simulink model "servo_hub_task_sys"  (R2023a)
settings: Solver=FixedStepDiscrete  StartTime=0.0  StopTime=10.0  RelTol=1e-3
settings Model: Creator=Administrator  LastModifiedBy=Administrator

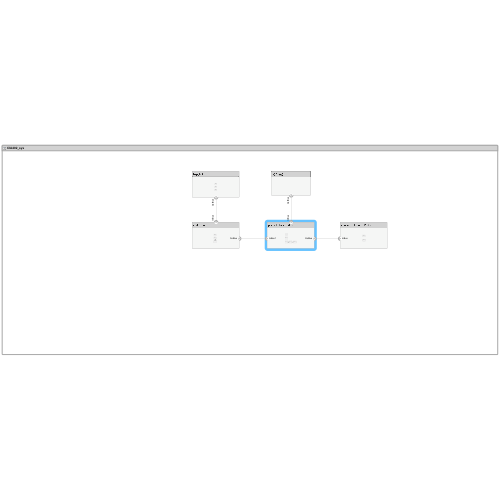
[thumbnail: Simulink's stored preview of the top-level diagram]
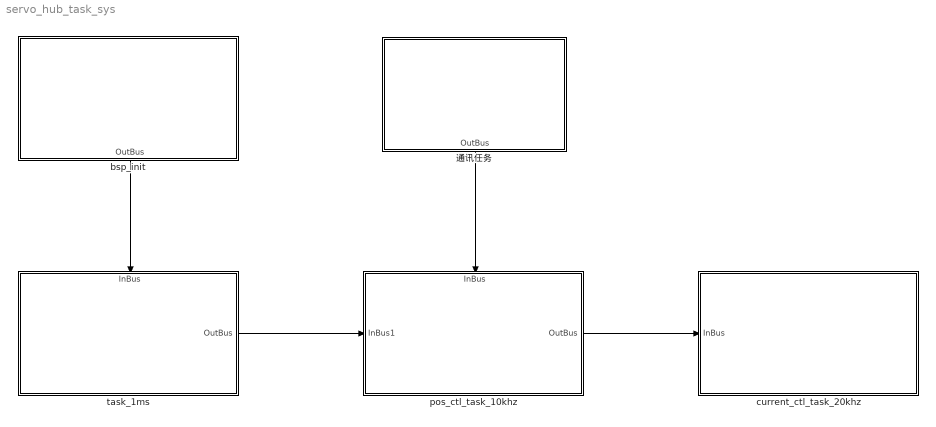
== system servo_hub_task_sys ==
  bsp_init : Subsystem
      settings: PortSchema="{\"entries\":[{\"content\":{\"headerSize\":26,\"margin\":15,\"minimumSpacing\":25,\"sides\":[{\"content\":{},\"type\":\"ConnectorPlacement.EquallySpacedRectSide\",\"uuid\":\"1beaa6a8-afd1-4db0-ba36-e52cb0b52ffd\"},{\"content\":{\"side\":\"RIGHT\"},\"type\":\"ConnectorPlacement.EquallySpacedRectSide\",\"uuid\":\"b483323e-58d5-432d-ab7d-aadce63dbe6f\"},{\"content\":{\"side\":\"TOP\"},\"type\":\"ConnectorPlacement.EquallySpacedRectSide\",\"uuid\":\"9aa6bb67-c79d-4421-a771-0f032b496522\"},{\"content\":{\"connectorIds\":[\"Out1\"],\"side\":\"BOTTOM\"},\"type\":\"ConnectorPlacement.EquallySpacedRectSide\",\"uuid\":\"df1d6553-7fe8-4c19-b309-8013b66b66f3\"}]},\"type\":\"ConnectorPlacement.EquallySpacedConnector\",\"uuid\":\"06545d34-e2f8-440d-8858-488d7d5d7ce4\"}],\"packageUris\":[\"http://schema.mathworks.com/mf0/Connector/R2020b\"],\"version\":\"1.0\"}"
  current_ctl_task_20khz : Subsystem
      settings: PortSchema="{\"entries\":[{\"content\":{\"headerSize\":26,\"margin\":15,\"minimumSpacing\":25,\"sides\":[{\"content\":{\"connectorIds\":[\"In1\"]},\"type\":\"ConnectorPlacement.EquallySpacedRectSide\",\"uuid\":\"1beaa6a8-afd1-4db0-ba36-e52cb0b52ffd\"},{\"content\":{\"side\":\"RIGHT\"},\"type\":\"ConnectorPlacement.EquallySpacedRectSide\",\"uuid\":\"b483323e-58d5-432d-ab7d-aadce63dbe6f\"},{\"content\":{\"side\":\"TOP\"},\"type\":\"ConnectorPlacement.EquallySpacedRectSide\",\"uuid\":\"9aa6bb67-c79d-4421-a771-0f032b496522\"}]},\"type\":\"ConnectorPlacement.EquallySpacedConnector\",\"uuid\":\"06545d34-e2f8-440d-8858-488d7d5d7ce4\"}],\"packageUris\":[\"http://schema.mathworks.com/mf0/Connector/R2020b\"],\"version\":\"1.0\"}"
  pos_ctl_task_10khz : Subsystem
      settings: PortSchema="{\"entries\":[{\"content\":{\"headerSize\":26,\"margin\":15,\"minimumSpacing\":25,\"sides\":[{\"content\":{\"connectorIds\":[\"In1\"]},\"type\":\"ConnectorPlacement.EquallySpacedRectSide\",\"uuid\":\"1beaa6a8-afd1-4db0-ba36-e52cb0b52ffd\"},{\"content\":{\"connectorIds\":[\"Out1\"],\"side\":\"RIGHT\"},\"type\":\"ConnectorPlacement.EquallySpacedRectSide\",\"uuid\":\"b483323e-58d5-432d-ab7d-aadce63dbe6f\"},{\"content\":{\"connectorIds\":[\"In2\"],\"side\":\"TOP\"},\"type\":\"ConnectorPlacement.EquallySpacedRectSide\",\"uuid\":\"9aa6bb67-c79d-4421-a771-0f032b496522\"}]},\"type\":\"ConnectorPlacement.EquallySpacedConnector\",\"uuid\":\"06545d34-e2f8-440d-8858-488d7d5d7ce4\"}],\"packageUris\":[\"http://schema.mathworks.com/mf0/Connector/R2020b\"],\"version\":\"1.0\"}"
  task_1ms : Subsystem
      settings: PortSchema="{\"entries\":[{\"content\":{\"headerSize\":26,\"margin\":15,\"minimumSpacing\":25,\"sides\":[{\"content\":{},\"type\":\"ConnectorPlacement.EquallySpacedRectSide\",\"uuid\":\"1beaa6a8-afd1-4db0-ba36-e52cb0b52ffd\"},{\"content\":{\"connectorIds\":[\"Out1\"],\"side\":\"RIGHT\"},\"type\":\"ConnectorPlacement.EquallySpacedRectSide\",\"uuid\":\"b483323e-58d5-432d-ab7d-aadce63dbe6f\"},{\"content\":{\"connectorIds\":[\"In1\"],\"side\":\"TOP\"},\"type\":\"ConnectorPlacement.EquallySpacedRectSide\",\"uuid\":\"9aa6bb67-c79d-4421-a771-0f032b496522\"}]},\"type\":\"ConnectorPlacement.EquallySpacedConnector\",\"uuid\":\"06545d34-e2f8-440d-8858-488d7d5d7ce4\"}],\"packageUris\":[\"http://schema.mathworks.com/mf0/Connector/R2020b\"],\"version\":\"1.0\"}"
  通讯任务 : Subsystem
      settings: PortSchema="{\"entries\":[{\"content\":{\"headerSize\":26,\"margin\":15,\"minimumSpacing\":25,\"sides\":[{\"content\":{},\"type\":\"ConnectorPlacement.EquallySpacedRectSide\",\"uuid\":\"1beaa6a8-afd1-4db0-ba36-e52cb0b52ffd\"},{\"content\":{\"side\":\"RIGHT\"},\"type\":\"ConnectorPlacement.EquallySpacedRectSide\",\"uuid\":\"b483323e-58d5-432d-ab7d-aadce63dbe6f\"},{\"content\":{\"side\":\"TOP\"},\"type\":\"ConnectorPlacement.EquallySpacedRectSide\",\"uuid\":\"9aa6bb67-c79d-4421-a771-0f032b496522\"},{\"content\":{\"connectorIds\":[\"Out1\"],\"side\":\"BOTTOM\"},\"type\":\"ConnectorPlacement.EquallySpacedRectSide\",\"uuid\":\"0c5aa3c4-d775-46bd-bbd0-0799f29f5e5b\"}]},\"type\":\"ConnectorPlacement.EquallySpacedConnector\",\"uuid\":\"06545d34-e2f8-440d-8858-488d7d5d7ce4\"}],\"packageUris\":[\"http://schema.mathworks.com/mf0/Connector/R2020b\"],\"version\":\"1.0\"}"
  wires:
  bsp_init/1(OutBus) -> task_1ms/1(InBus)
  pos_ctl_task_10khz/1(OutBus) -> current_ctl_task_20khz/1(InBus)
  通讯任务/1(OutBus) -> pos_ctl_task_10khz/2(InBus)
  task_1ms/1(OutBus) -> pos_ctl_task_10khz/1(InBus1)

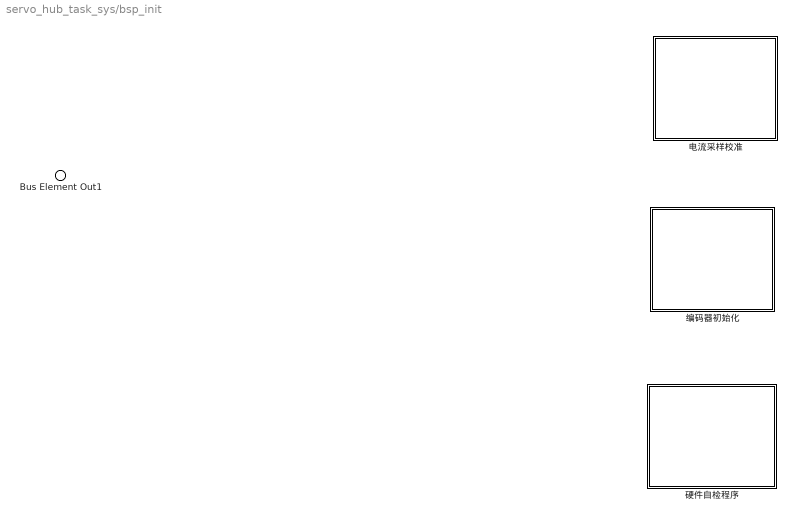
== system servo_hub_task_sys/bsp_init ==
  电流采样校准 : Subsystem
      settings: PortSchema="{\"entries\":[{\"content\":{\"headerSize\":26,\"margin\":15,\"minimumSpacing\":25,\"sides\":[{\"content\":{},\"type\":\"ConnectorPlacement.EquallySpacedRectSide\",\"uuid\":\"1beaa6a8-afd1-4db0-ba36-e52cb0b52ffd\"},{\"content\":{\"side\":\"RIGHT\"},\"type\":\"ConnectorPlacement.EquallySpacedRectSide\",\"uuid\":\"b483323e-58d5-432d-ab7d-aadce63dbe6f\"},{\"content\":{\"side\":\"TOP\"},\"type\":\"ConnectorPlacement.EquallySpacedRectSide\",\"uuid\":\"9aa6bb67-c79d-4421-a771-0f032b496522\"}]},\"type\":\"ConnectorPlacement.EquallySpacedConnector\",\"uuid\":\"06545d34-e2f8-440d-8858-488d7d5d7ce4\"}],\"packageUris\":[\"http://schema.mathworks.com/mf0/Connector/R2020b\"],\"version\":\"1.0\"}"
  硬件自检程序 : Subsystem
      settings: PortSchema="{\"entries\":[{\"content\":{\"headerSize\":26,\"margin\":15,\"minimumSpacing\":25,\"sides\":[{\"content\":{},\"type\":\"ConnectorPlacement.EquallySpacedRectSide\",\"uuid\":\"1beaa6a8-afd1-4db0-ba36-e52cb0b52ffd\"},{\"content\":{\"side\":\"RIGHT\"},\"type\":\"ConnectorPlacement.EquallySpacedRectSide\",\"uuid\":\"b483323e-58d5-432d-ab7d-aadce63dbe6f\"},{\"content\":{\"side\":\"TOP\"},\"type\":\"ConnectorPlacement.EquallySpacedRectSide\",\"uuid\":\"9aa6bb67-c79d-4421-a771-0f032b496522\"}]},\"type\":\"ConnectorPlacement.EquallySpacedConnector\",\"uuid\":\"06545d34-e2f8-440d-8858-488d7d5d7ce4\"}],\"packageUris\":[\"http://schema.mathworks.com/mf0/Connector/R2020b\"],\"version\":\"1.0\"}"
  编码器初始化 : Subsystem
      settings: PortSchema="{\"entries\":[{\"content\":{\"headerSize\":26,\"margin\":15,\"minimumSpacing\":25,\"sides\":[{\"content\":{},\"type\":\"ConnectorPlacement.EquallySpacedRectSide\",\"uuid\":\"1beaa6a8-afd1-4db0-ba36-e52cb0b52ffd\"},{\"content\":{\"side\":\"RIGHT\"},\"type\":\"ConnectorPlacement.EquallySpacedRectSide\",\"uuid\":\"b483323e-58d5-432d-ab7d-aadce63dbe6f\"},{\"content\":{\"side\":\"TOP\"},\"type\":\"ConnectorPlacement.EquallySpacedRectSide\",\"uuid\":\"9aa6bb67-c79d-4421-a771-0f032b496522\"}]},\"type\":\"ConnectorPlacement.EquallySpacedConnector\",\"uuid\":\"06545d34-e2f8-440d-8858-488d7d5d7ce4\"}],\"packageUris\":[\"http://schema.mathworks.com/mf0/Connector/R2020b\"],\"version\":\"1.0\"}"
  Bus Element Out1 : Outport  PortName=OutBus

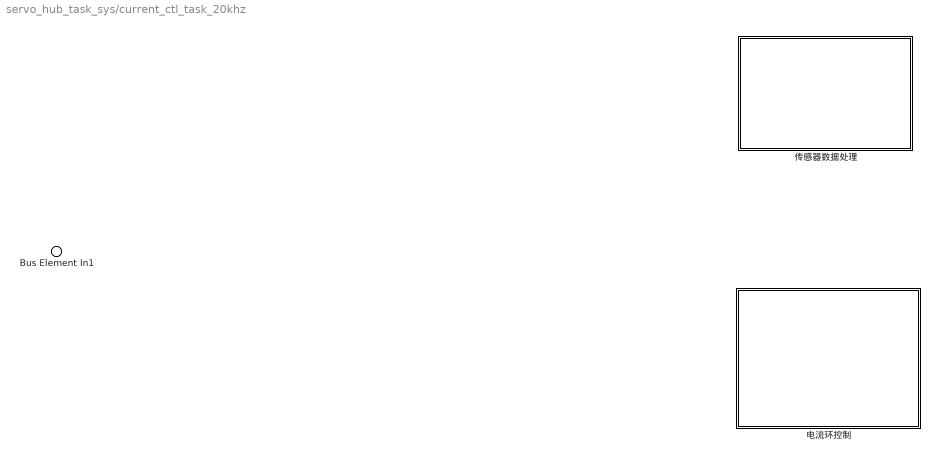
== system servo_hub_task_sys/current_ctl_task_20khz ==
  Bus Element In1 : Inport  PortName=InBus
  传感器数据处理 : Subsystem
      settings: PortSchema="{\"entries\":[{\"content\":{\"headerSize\":26,\"margin\":15,\"minimumSpacing\":25,\"sides\":[{\"content\":{},\"type\":\"ConnectorPlacement.EquallySpacedRectSide\",\"uuid\":\"1beaa6a8-afd1-4db0-ba36-e52cb0b52ffd\"},{\"content\":{\"side\":\"RIGHT\"},\"type\":\"ConnectorPlacement.EquallySpacedRectSide\",\"uuid\":\"b483323e-58d5-432d-ab7d-aadce63dbe6f\"},{\"content\":{\"side\":\"TOP\"},\"type\":\"ConnectorPlacement.EquallySpacedRectSide\",\"uuid\":\"9aa6bb67-c79d-4421-a771-0f032b496522\"}]},\"type\":\"ConnectorPlacement.EquallySpacedConnector\",\"uuid\":\"06545d34-e2f8-440d-8858-488d7d5d7ce4\"}],\"packageUris\":[\"http://schema.mathworks.com/mf0/Connector/R2020b\"],\"version\":\"1.0\"}"
  电流环控制 : Subsystem
      settings: PortSchema="{\"entries\":[{\"content\":{\"headerSize\":26,\"margin\":15,\"minimumSpacing\":25,\"sides\":[{\"content\":{},\"type\":\"ConnectorPlacement.EquallySpacedRectSide\",\"uuid\":\"1beaa6a8-afd1-4db0-ba36-e52cb0b52ffd\"},{\"content\":{\"side\":\"RIGHT\"},\"type\":\"ConnectorPlacement.EquallySpacedRectSide\",\"uuid\":\"b483323e-58d5-432d-ab7d-aadce63dbe6f\"},{\"content\":{\"side\":\"TOP\"},\"type\":\"ConnectorPlacement.EquallySpacedRectSide\",\"uuid\":\"9aa6bb67-c79d-4421-a771-0f032b496522\"}]},\"type\":\"ConnectorPlacement.EquallySpacedConnector\",\"uuid\":\"06545d34-e2f8-440d-8858-488d7d5d7ce4\"}],\"packageUris\":[\"http://schema.mathworks.com/mf0/Connector/R2020b\"],\"version\":\"1.0\"}"

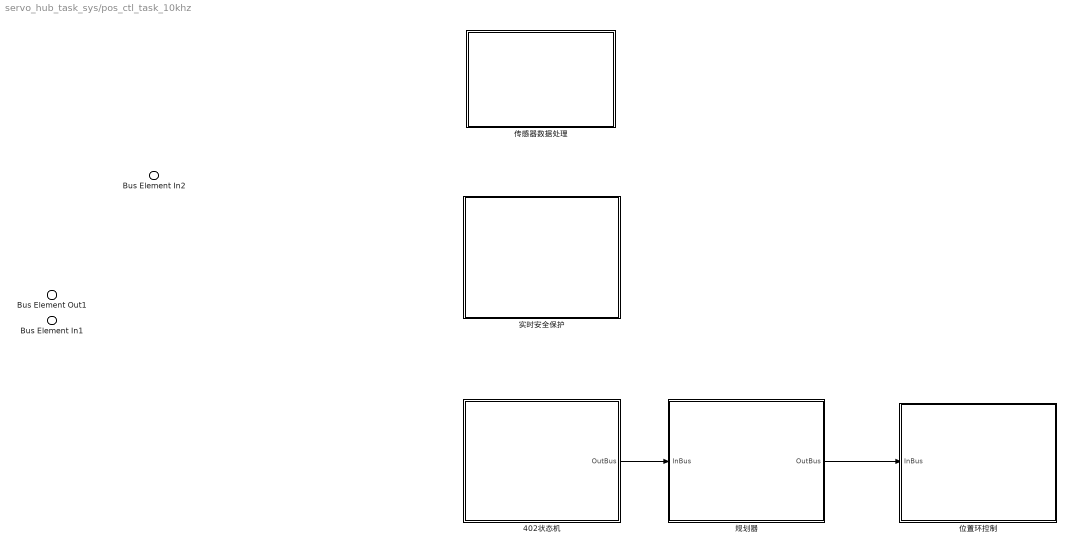
== system servo_hub_task_sys/pos_ctl_task_10khz ==
  Bus Element In2 : Inport  PortName=InBus1
  Bus Element In1 : Inport  Port=2  PortName=InBus
  402状态机 : Subsystem
      settings: PortSchema="{\"entries\":[{\"content\":{\"headerSize\":26,\"margin\":15,\"minimumSpacing\":25,\"sides\":[{\"content\":{},\"type\":\"ConnectorPlacement.EquallySpacedRectSide\",\"uuid\":\"1beaa6a8-afd1-4db0-ba36-e52cb0b52ffd\"},{\"content\":{\"connectorIds\":[\"Out1\"],\"side\":\"RIGHT\"},\"type\":\"ConnectorPlacement.EquallySpacedRectSide\",\"uuid\":\"b483323e-58d5-432d-ab7d-aadce63dbe6f\"},{\"content\":{\"side\":\"TOP\"},\"type\":\"ConnectorPlacement.EquallySpacedRectSide\",\"uuid\":\"9aa6bb67-c79d-4421-a771-0f032b496522\"}]},\"type\":\"ConnectorPlacement.EquallySpacedConnector\",\"uuid\":\"06545d34-e2f8-440d-8858-488d7d5d7ce4\"}],\"packageUris\":[\"http://schema.mathworks.com/mf0/Connector/R2020b\"],\"version\":\"1.0\"}"
  传感器数据处理 : Subsystem
      settings: PortSchema="{\"entries\":[{\"content\":{\"headerSize\":26,\"margin\":15,\"minimumSpacing\":25,\"sides\":[{\"content\":{},\"type\":\"ConnectorPlacement.EquallySpacedRectSide\",\"uuid\":\"1beaa6a8-afd1-4db0-ba36-e52cb0b52ffd\"},{\"content\":{\"side\":\"RIGHT\"},\"type\":\"ConnectorPlacement.EquallySpacedRectSide\",\"uuid\":\"b483323e-58d5-432d-ab7d-aadce63dbe6f\"},{\"content\":{\"side\":\"TOP\"},\"type\":\"ConnectorPlacement.EquallySpacedRectSide\",\"uuid\":\"9aa6bb67-c79d-4421-a771-0f032b496522\"}]},\"type\":\"ConnectorPlacement.EquallySpacedConnector\",\"uuid\":\"06545d34-e2f8-440d-8858-488d7d5d7ce4\"}],\"packageUris\":[\"http://schema.mathworks.com/mf0/Connector/R2020b\"],\"version\":\"1.0\"}"
  位置环控制 : Subsystem
      settings: PortSchema="{\"entries\":[{\"content\":{\"headerSize\":26,\"margin\":15,\"minimumSpacing\":25,\"sides\":[{\"content\":{\"connectorIds\":[\"In1\"]},\"type\":\"ConnectorPlacement.EquallySpacedRectSide\",\"uuid\":\"1beaa6a8-afd1-4db0-ba36-e52cb0b52ffd\"},{\"content\":{\"side\":\"RIGHT\"},\"type\":\"ConnectorPlacement.EquallySpacedRectSide\",\"uuid\":\"b483323e-58d5-432d-ab7d-aadce63dbe6f\"},{\"content\":{\"side\":\"TOP\"},\"type\":\"ConnectorPlacement.EquallySpacedRectSide\",\"uuid\":\"9aa6bb67-c79d-4421-a771-0f032b496522\"}]},\"type\":\"ConnectorPlacement.EquallySpacedConnector\",\"uuid\":\"06545d34-e2f8-440d-8858-488d7d5d7ce4\"}],\"packageUris\":[\"http://schema.mathworks.com/mf0/Connector/R2020b\"],\"version\":\"1.0\"}"
  实时安全保护 : Subsystem
      settings: PortSchema="{\"entries\":[{\"content\":{\"headerSize\":26,\"margin\":15,\"minimumSpacing\":25,\"sides\":[{\"content\":{},\"type\":\"ConnectorPlacement.EquallySpacedRectSide\",\"uuid\":\"1beaa6a8-afd1-4db0-ba36-e52cb0b52ffd\"},{\"content\":{\"side\":\"RIGHT\"},\"type\":\"ConnectorPlacement.EquallySpacedRectSide\",\"uuid\":\"b483323e-58d5-432d-ab7d-aadce63dbe6f\"},{\"content\":{\"side\":\"TOP\"},\"type\":\"ConnectorPlacement.EquallySpacedRectSide\",\"uuid\":\"9aa6bb67-c79d-4421-a771-0f032b496522\"}]},\"type\":\"ConnectorPlacement.EquallySpacedConnector\",\"uuid\":\"06545d34-e2f8-440d-8858-488d7d5d7ce4\"}],\"packageUris\":[\"http://schema.mathworks.com/mf0/Connector/R2020b\"],\"version\":\"1.0\"}"
  规划器 : Subsystem
      settings: PortSchema="{\"entries\":[{\"content\":{\"headerSize\":26,\"margin\":15,\"minimumSpacing\":25,\"sides\":[{\"content\":{\"connectorIds\":[\"In1\"]},\"type\":\"ConnectorPlacement.EquallySpacedRectSide\",\"uuid\":\"1beaa6a8-afd1-4db0-ba36-e52cb0b52ffd\"},{\"content\":{\"connectorIds\":[\"Out1\"],\"side\":\"RIGHT\"},\"type\":\"ConnectorPlacement.EquallySpacedRectSide\",\"uuid\":\"b483323e-58d5-432d-ab7d-aadce63dbe6f\"},{\"content\":{\"side\":\"TOP\"},\"type\":\"ConnectorPlacement.EquallySpacedRectSide\",\"uuid\":\"9aa6bb67-c79d-4421-a771-0f032b496522\"}]},\"type\":\"ConnectorPlacement.EquallySpacedConnector\",\"uuid\":\"06545d34-e2f8-440d-8858-488d7d5d7ce4\"}],\"packageUris\":[\"http://schema.mathworks.com/mf0/Connector/R2020b\"],\"version\":\"1.0\"}"
  Bus Element Out1 : Outport  PortName=OutBus
  wires:
  402状态机/1(OutBus) -> 规划器/1(InBus)
  规划器/1(OutBus) -> 位置环控制/1(InBus)

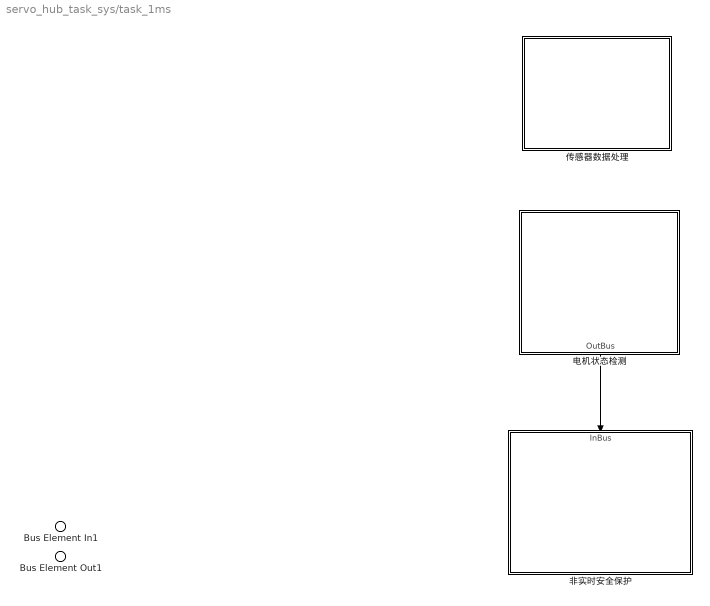
== system servo_hub_task_sys/task_1ms ==
  Bus Element In1 : Inport  PortName=InBus
  传感器数据处理 : Subsystem
      settings: PortSchema="{\"entries\":[{\"content\":{\"headerSize\":26,\"margin\":15,\"minimumSpacing\":25,\"sides\":[{\"content\":{},\"type\":\"ConnectorPlacement.EquallySpacedRectSide\",\"uuid\":\"1beaa6a8-afd1-4db0-ba36-e52cb0b52ffd\"},{\"content\":{\"side\":\"RIGHT\"},\"type\":\"ConnectorPlacement.EquallySpacedRectSide\",\"uuid\":\"b483323e-58d5-432d-ab7d-aadce63dbe6f\"},{\"content\":{\"side\":\"TOP\"},\"type\":\"ConnectorPlacement.EquallySpacedRectSide\",\"uuid\":\"9aa6bb67-c79d-4421-a771-0f032b496522\"}]},\"type\":\"ConnectorPlacement.EquallySpacedConnector\",\"uuid\":\"06545d34-e2f8-440d-8858-488d7d5d7ce4\"}],\"packageUris\":[\"http://schema.mathworks.com/mf0/Connector/R2020b\"],\"version\":\"1.0\"}"
  电机状态检测 : Subsystem
      settings: PortSchema="{\"entries\":[{\"content\":{\"headerSize\":26,\"margin\":15,\"minimumSpacing\":25,\"sides\":[{\"content\":{},\"type\":\"ConnectorPlacement.EquallySpacedRectSide\",\"uuid\":\"1beaa6a8-afd1-4db0-ba36-e52cb0b52ffd\"},{\"content\":{\"side\":\"RIGHT\"},\"type\":\"ConnectorPlacement.EquallySpacedRectSide\",\"uuid\":\"b483323e-58d5-432d-ab7d-aadce63dbe6f\"},{\"content\":{\"side\":\"TOP\"},\"type\":\"ConnectorPlacement.EquallySpacedRectSide\",\"uuid\":\"9aa6bb67-c79d-4421-a771-0f032b496522\"},{\"content\":{\"connectorIds\":[\"Out1\"],\"side\":\"BOTTOM\"},\"type\":\"ConnectorPlacement.EquallySpacedRectSide\",\"uuid\":\"f74b369b-1106-4e9b-b41f-5530fa0be2a4\"}]},\"type\":\"ConnectorPlacement.EquallySpacedConnector\",\"uuid\":\"06545d34-e2f8-440d-8858-488d7d5d7ce4\"}],\"packageUris\":[\"http://schema.mathworks.com/mf0/Connector/R2020b\"],\"version\":\"1.0\"}"
  非实时安全保护 : Subsystem
      settings: PortSchema="{\"entries\":[{\"content\":{\"headerSize\":26,\"margin\":15,\"minimumSpacing\":25,\"sides\":[{\"content\":{},\"type\":\"ConnectorPlacement.EquallySpacedRectSide\",\"uuid\":\"1beaa6a8-afd1-4db0-ba36-e52cb0b52ffd\"},{\"content\":{\"side\":\"RIGHT\"},\"type\":\"ConnectorPlacement.EquallySpacedRectSide\",\"uuid\":\"b483323e-58d5-432d-ab7d-aadce63dbe6f\"},{\"content\":{\"connectorIds\":[\"In1\"],\"side\":\"TOP\"},\"type\":\"ConnectorPlacement.EquallySpacedRectSide\",\"uuid\":\"9aa6bb67-c79d-4421-a771-0f032b496522\"}]},\"type\":\"ConnectorPlacement.EquallySpacedConnector\",\"uuid\":\"06545d34-e2f8-440d-8858-488d7d5d7ce4\"}],\"packageUris\":[\"http://schema.mathworks.com/mf0/Connector/R2020b\"],\"version\":\"1.0\"}"
  Bus Element Out1 : Outport  PortName=OutBus
  wires:
  电机状态检测/1(OutBus) -> 非实时安全保护/1(InBus)

== system servo_hub_task_sys/通讯任务 ==
  Bus Element Out1 : Outport  PortName=OutBus

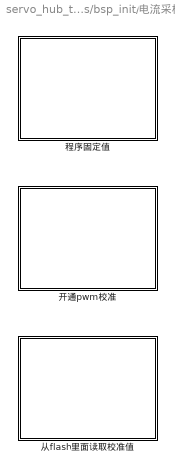
== system servo_hub_task_sys/bsp_init/电流采样校准 ==
  从flash里面读取校准值 : Subsystem
      settings: PortSchema="{\"entries\":[{\"content\":{\"headerSize\":26,\"margin\":15,\"minimumSpacing\":25,\"sides\":[{\"content\":{},\"type\":\"ConnectorPlacement.EquallySpacedRectSide\",\"uuid\":\"1beaa6a8-afd1-4db0-ba36-e52cb0b52ffd\"},{\"content\":{\"side\":\"RIGHT\"},\"type\":\"ConnectorPlacement.EquallySpacedRectSide\",\"uuid\":\"b483323e-58d5-432d-ab7d-aadce63dbe6f\"},{\"content\":{\"side\":\"TOP\"},\"type\":\"ConnectorPlacement.EquallySpacedRectSide\",\"uuid\":\"9aa6bb67-c79d-4421-a771-0f032b496522\"}]},\"type\":\"ConnectorPlacement.EquallySpacedConnector\",\"uuid\":\"06545d34-e2f8-440d-8858-488d7d5d7ce4\"}],\"packageUris\":[\"http://schema.mathworks.com/mf0/Connector/R2020b\"],\"version\":\"1.0\"}"
  开通pwm校准 : Subsystem
      settings: PortSchema="{\"entries\":[{\"content\":{\"headerSize\":26,\"margin\":15,\"minimumSpacing\":25,\"sides\":[{\"content\":{},\"type\":\"ConnectorPlacement.EquallySpacedRectSide\",\"uuid\":\"1beaa6a8-afd1-4db0-ba36-e52cb0b52ffd\"},{\"content\":{\"side\":\"RIGHT\"},\"type\":\"ConnectorPlacement.EquallySpacedRectSide\",\"uuid\":\"b483323e-58d5-432d-ab7d-aadce63dbe6f\"},{\"content\":{\"side\":\"TOP\"},\"type\":\"ConnectorPlacement.EquallySpacedRectSide\",\"uuid\":\"9aa6bb67-c79d-4421-a771-0f032b496522\"}]},\"type\":\"ConnectorPlacement.EquallySpacedConnector\",\"uuid\":\"06545d34-e2f8-440d-8858-488d7d5d7ce4\"}],\"packageUris\":[\"http://schema.mathworks.com/mf0/Connector/R2020b\"],\"version\":\"1.0\"}"
  程序固定值 : Subsystem
      settings: PortSchema="{\"entries\":[{\"content\":{\"headerSize\":26,\"margin\":15,\"minimumSpacing\":25,\"sides\":[{\"content\":{},\"type\":\"ConnectorPlacement.EquallySpacedRectSide\",\"uuid\":\"1beaa6a8-afd1-4db0-ba36-e52cb0b52ffd\"},{\"content\":{\"side\":\"RIGHT\"},\"type\":\"ConnectorPlacement.EquallySpacedRectSide\",\"uuid\":\"b483323e-58d5-432d-ab7d-aadce63dbe6f\"},{\"content\":{\"side\":\"TOP\"},\"type\":\"ConnectorPlacement.EquallySpacedRectSide\",\"uuid\":\"9aa6bb67-c79d-4421-a771-0f032b496522\"}]},\"type\":\"ConnectorPlacement.EquallySpacedConnector\",\"uuid\":\"06545d34-e2f8-440d-8858-488d7d5d7ce4\"}],\"packageUris\":[\"http://schema.mathworks.com/mf0/Connector/R2020b\"],\"version\":\"1.0\"}"

== system servo_hub_task_sys/bsp_init/硬件自检程序 ==

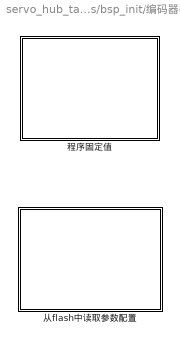
== system servo_hub_task_sys/bsp_init/编码器初始化 ==
  从flash中读取参数配置 : Subsystem
      settings: PortSchema="{\"entries\":[{\"content\":{\"headerSize\":26,\"margin\":15,\"minimumSpacing\":25,\"sides\":[{\"content\":{},\"type\":\"ConnectorPlacement.EquallySpacedRectSide\",\"uuid\":\"1beaa6a8-afd1-4db0-ba36-e52cb0b52ffd\"},{\"content\":{\"side\":\"RIGHT\"},\"type\":\"ConnectorPlacement.EquallySpacedRectSide\",\"uuid\":\"b483323e-58d5-432d-ab7d-aadce63dbe6f\"},{\"content\":{\"side\":\"TOP\"},\"type\":\"ConnectorPlacement.EquallySpacedRectSide\",\"uuid\":\"9aa6bb67-c79d-4421-a771-0f032b496522\"}]},\"type\":\"ConnectorPlacement.EquallySpacedConnector\",\"uuid\":\"06545d34-e2f8-440d-8858-488d7d5d7ce4\"}],\"packageUris\":[\"http://schema.mathworks.com/mf0/Connector/R2020b\"],\"version\":\"1.0\"}"
  程序固定值 : Subsystem
      settings: PortSchema="{\"entries\":[{\"content\":{\"headerSize\":26,\"margin\":15,\"minimumSpacing\":25,\"sides\":[{\"content\":{},\"type\":\"ConnectorPlacement.EquallySpacedRectSide\",\"uuid\":\"1beaa6a8-afd1-4db0-ba36-e52cb0b52ffd\"},{\"content\":{\"side\":\"RIGHT\"},\"type\":\"ConnectorPlacement.EquallySpacedRectSide\",\"uuid\":\"b483323e-58d5-432d-ab7d-aadce63dbe6f\"},{\"content\":{\"side\":\"TOP\"},\"type\":\"ConnectorPlacement.EquallySpacedRectSide\",\"uuid\":\"9aa6bb67-c79d-4421-a771-0f032b496522\"}]},\"type\":\"ConnectorPlacement.EquallySpacedConnector\",\"uuid\":\"06545d34-e2f8-440d-8858-488d7d5d7ce4\"}],\"packageUris\":[\"http://schema.mathworks.com/mf0/Connector/R2020b\"],\"version\":\"1.0\"}"

== system servo_hub_task_sys/current_ctl_task_20khz/传感器数据处理 ==

== system servo_hub_task_sys/current_ctl_task_20khz/电流环控制 ==

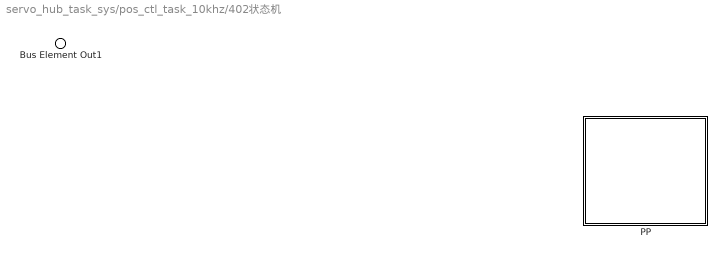
== system servo_hub_task_sys/pos_ctl_task_10khz/402状态机 ==
  PP : Subsystem
      settings: PortSchema="{\"entries\":[{\"content\":{\"headerSize\":26,\"margin\":15,\"minimumSpacing\":25,\"sides\":[{\"content\":{},\"type\":\"ConnectorPlacement.EquallySpacedRectSide\",\"uuid\":\"1beaa6a8-afd1-4db0-ba36-e52cb0b52ffd\"},{\"content\":{\"side\":\"RIGHT\"},\"type\":\"ConnectorPlacement.EquallySpacedRectSide\",\"uuid\":\"b483323e-58d5-432d-ab7d-aadce63dbe6f\"},{\"content\":{\"side\":\"TOP\"},\"type\":\"ConnectorPlacement.EquallySpacedRectSide\",\"uuid\":\"9aa6bb67-c79d-4421-a771-0f032b496522\"}]},\"type\":\"ConnectorPlacement.EquallySpacedConnector\",\"uuid\":\"06545d34-e2f8-440d-8858-488d7d5d7ce4\"}],\"packageUris\":[\"http://schema.mathworks.com/mf0/Connector/R2020b\"],\"version\":\"1.0\"}"
  Bus Element Out1 : Outport  PortName=OutBus

== system servo_hub_task_sys/pos_ctl_task_10khz/传感器数据处理 ==

== system servo_hub_task_sys/pos_ctl_task_10khz/位置环控制 ==
  Bus Element In1 : Inport  PortName=InBus

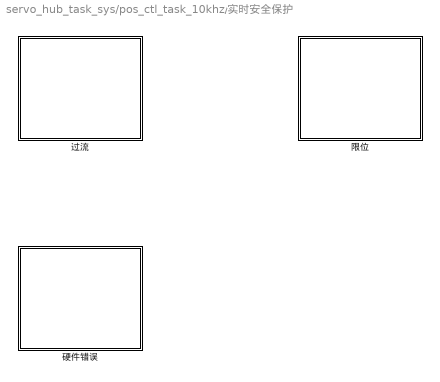
== system servo_hub_task_sys/pos_ctl_task_10khz/实时安全保护 ==
  硬件错误 : Subsystem
      settings: PortSchema="{\"entries\":[{\"content\":{\"headerSize\":26,\"margin\":15,\"minimumSpacing\":25,\"sides\":[{\"content\":{},\"type\":\"ConnectorPlacement.EquallySpacedRectSide\",\"uuid\":\"1beaa6a8-afd1-4db0-ba36-e52cb0b52ffd\"},{\"content\":{\"side\":\"RIGHT\"},\"type\":\"ConnectorPlacement.EquallySpacedRectSide\",\"uuid\":\"b483323e-58d5-432d-ab7d-aadce63dbe6f\"},{\"content\":{\"side\":\"TOP\"},\"type\":\"ConnectorPlacement.EquallySpacedRectSide\",\"uuid\":\"9aa6bb67-c79d-4421-a771-0f032b496522\"}]},\"type\":\"ConnectorPlacement.EquallySpacedConnector\",\"uuid\":\"06545d34-e2f8-440d-8858-488d7d5d7ce4\"}],\"packageUris\":[\"http://schema.mathworks.com/mf0/Connector/R2020b\"],\"version\":\"1.0\"}"
  过流 : Subsystem
      settings: PortSchema="{\"entries\":[{\"content\":{\"headerSize\":26,\"margin\":15,\"minimumSpacing\":25,\"sides\":[{\"content\":{},\"type\":\"ConnectorPlacement.EquallySpacedRectSide\",\"uuid\":\"1beaa6a8-afd1-4db0-ba36-e52cb0b52ffd\"},{\"content\":{\"side\":\"RIGHT\"},\"type\":\"ConnectorPlacement.EquallySpacedRectSide\",\"uuid\":\"b483323e-58d5-432d-ab7d-aadce63dbe6f\"},{\"content\":{\"side\":\"TOP\"},\"type\":\"ConnectorPlacement.EquallySpacedRectSide\",\"uuid\":\"9aa6bb67-c79d-4421-a771-0f032b496522\"}]},\"type\":\"ConnectorPlacement.EquallySpacedConnector\",\"uuid\":\"06545d34-e2f8-440d-8858-488d7d5d7ce4\"}],\"packageUris\":[\"http://schema.mathworks.com/mf0/Connector/R2020b\"],\"version\":\"1.0\"}"
  限位 : Subsystem
      settings: PortSchema="{\"entries\":[{\"content\":{\"headerSize\":26,\"margin\":15,\"minimumSpacing\":25,\"sides\":[{\"content\":{},\"type\":\"ConnectorPlacement.EquallySpacedRectSide\",\"uuid\":\"1beaa6a8-afd1-4db0-ba36-e52cb0b52ffd\"},{\"content\":{\"side\":\"RIGHT\"},\"type\":\"ConnectorPlacement.EquallySpacedRectSide\",\"uuid\":\"b483323e-58d5-432d-ab7d-aadce63dbe6f\"},{\"content\":{\"side\":\"TOP\"},\"type\":\"ConnectorPlacement.EquallySpacedRectSide\",\"uuid\":\"9aa6bb67-c79d-4421-a771-0f032b496522\"}]},\"type\":\"ConnectorPlacement.EquallySpacedConnector\",\"uuid\":\"06545d34-e2f8-440d-8858-488d7d5d7ce4\"}],\"packageUris\":[\"http://schema.mathworks.com/mf0/Connector/R2020b\"],\"version\":\"1.0\"}"

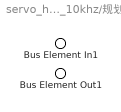
== system servo_hub_task_sys/pos_ctl_task_10khz/规划器 ==
  Bus Element In1 : Inport  PortName=InBus
  Bus Element Out1 : Outport  PortName=OutBus

== system servo_hub_task_sys/task_1ms/传感器数据处理 ==

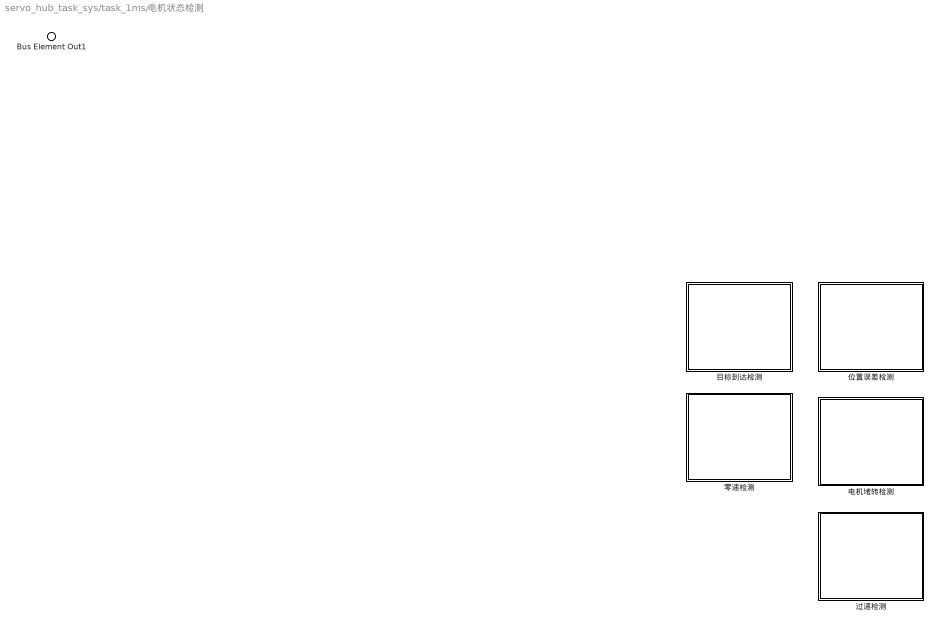
== system servo_hub_task_sys/task_1ms/电机状态检测 ==
  位置误差检测 : Subsystem
      settings: PortSchema="{\"entries\":[{\"content\":{\"headerSize\":26,\"margin\":15,\"minimumSpacing\":25,\"sides\":[{\"content\":{},\"type\":\"ConnectorPlacement.EquallySpacedRectSide\",\"uuid\":\"1beaa6a8-afd1-4db0-ba36-e52cb0b52ffd\"},{\"content\":{\"side\":\"RIGHT\"},\"type\":\"ConnectorPlacement.EquallySpacedRectSide\",\"uuid\":\"b483323e-58d5-432d-ab7d-aadce63dbe6f\"},{\"content\":{\"side\":\"TOP\"},\"type\":\"ConnectorPlacement.EquallySpacedRectSide\",\"uuid\":\"9aa6bb67-c79d-4421-a771-0f032b496522\"}]},\"type\":\"ConnectorPlacement.EquallySpacedConnector\",\"uuid\":\"06545d34-e2f8-440d-8858-488d7d5d7ce4\"}],\"packageUris\":[\"http://schema.mathworks.com/mf0/Connector/R2020b\"],\"version\":\"1.0\"}"
  电机堵转检测 : Subsystem
      settings: PortSchema="{\"entries\":[{\"content\":{\"headerSize\":26,\"margin\":15,\"minimumSpacing\":25,\"sides\":[{\"content\":{},\"type\":\"ConnectorPlacement.EquallySpacedRectSide\",\"uuid\":\"1beaa6a8-afd1-4db0-ba36-e52cb0b52ffd\"},{\"content\":{\"side\":\"RIGHT\"},\"type\":\"ConnectorPlacement.EquallySpacedRectSide\",\"uuid\":\"b483323e-58d5-432d-ab7d-aadce63dbe6f\"},{\"content\":{\"side\":\"TOP\"},\"type\":\"ConnectorPlacement.EquallySpacedRectSide\",\"uuid\":\"9aa6bb67-c79d-4421-a771-0f032b496522\"}]},\"type\":\"ConnectorPlacement.EquallySpacedConnector\",\"uuid\":\"06545d34-e2f8-440d-8858-488d7d5d7ce4\"}],\"packageUris\":[\"http://schema.mathworks.com/mf0/Connector/R2020b\"],\"version\":\"1.0\"}"
  目标到达检测 : Subsystem
      settings: PortSchema="{\"entries\":[{\"content\":{\"headerSize\":26,\"margin\":15,\"minimumSpacing\":25,\"sides\":[{\"content\":{},\"type\":\"ConnectorPlacement.EquallySpacedRectSide\",\"uuid\":\"1beaa6a8-afd1-4db0-ba36-e52cb0b52ffd\"},{\"content\":{\"side\":\"RIGHT\"},\"type\":\"ConnectorPlacement.EquallySpacedRectSide\",\"uuid\":\"b483323e-58d5-432d-ab7d-aadce63dbe6f\"},{\"content\":{\"side\":\"TOP\"},\"type\":\"ConnectorPlacement.EquallySpacedRectSide\",\"uuid\":\"9aa6bb67-c79d-4421-a771-0f032b496522\"}]},\"type\":\"ConnectorPlacement.EquallySpacedConnector\",\"uuid\":\"06545d34-e2f8-440d-8858-488d7d5d7ce4\"}],\"packageUris\":[\"http://schema.mathworks.com/mf0/Connector/R2020b\"],\"version\":\"1.0\"}"
  过速检测 : Subsystem
      settings: PortSchema="{\"entries\":[{\"content\":{\"headerSize\":26,\"margin\":15,\"minimumSpacing\":25,\"sides\":[{\"content\":{},\"type\":\"ConnectorPlacement.EquallySpacedRectSide\",\"uuid\":\"1beaa6a8-afd1-4db0-ba36-e52cb0b52ffd\"},{\"content\":{\"side\":\"RIGHT\"},\"type\":\"ConnectorPlacement.EquallySpacedRectSide\",\"uuid\":\"b483323e-58d5-432d-ab7d-aadce63dbe6f\"},{\"content\":{\"side\":\"TOP\"},\"type\":\"ConnectorPlacement.EquallySpacedRectSide\",\"uuid\":\"9aa6bb67-c79d-4421-a771-0f032b496522\"}]},\"type\":\"ConnectorPlacement.EquallySpacedConnector\",\"uuid\":\"06545d34-e2f8-440d-8858-488d7d5d7ce4\"}],\"packageUris\":[\"http://schema.mathworks.com/mf0/Connector/R2020b\"],\"version\":\"1.0\"}"
  零速检测 : Subsystem
      settings: PortSchema="{\"entries\":[{\"content\":{\"headerSize\":26,\"margin\":15,\"minimumSpacing\":25,\"sides\":[{\"content\":{},\"type\":\"ConnectorPlacement.EquallySpacedRectSide\",\"uuid\":\"1beaa6a8-afd1-4db0-ba36-e52cb0b52ffd\"},{\"content\":{\"side\":\"RIGHT\"},\"type\":\"ConnectorPlacement.EquallySpacedRectSide\",\"uuid\":\"b483323e-58d5-432d-ab7d-aadce63dbe6f\"},{\"content\":{\"side\":\"TOP\"},\"type\":\"ConnectorPlacement.EquallySpacedRectSide\",\"uuid\":\"9aa6bb67-c79d-4421-a771-0f032b496522\"}]},\"type\":\"ConnectorPlacement.EquallySpacedConnector\",\"uuid\":\"06545d34-e2f8-440d-8858-488d7d5d7ce4\"}],\"packageUris\":[\"http://schema.mathworks.com/mf0/Connector/R2020b\"],\"version\":\"1.0\"}"
  Bus Element Out1 : Outport  PortName=OutBus

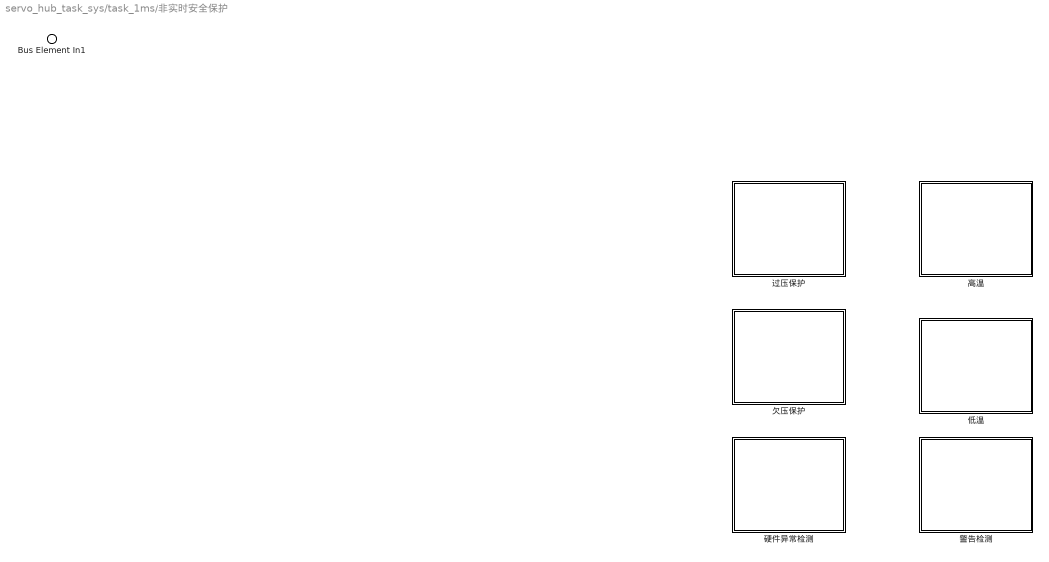
== system servo_hub_task_sys/task_1ms/非实时安全保护 ==
  Bus Element In1 : Inport  PortName=InBus
  低温 : Subsystem
      settings: PortSchema="{\"entries\":[{\"content\":{\"headerSize\":26,\"margin\":15,\"minimumSpacing\":25,\"sides\":[{\"content\":{},\"type\":\"ConnectorPlacement.EquallySpacedRectSide\",\"uuid\":\"1beaa6a8-afd1-4db0-ba36-e52cb0b52ffd\"},{\"content\":{\"side\":\"RIGHT\"},\"type\":\"ConnectorPlacement.EquallySpacedRectSide\",\"uuid\":\"b483323e-58d5-432d-ab7d-aadce63dbe6f\"},{\"content\":{\"side\":\"TOP\"},\"type\":\"ConnectorPlacement.EquallySpacedRectSide\",\"uuid\":\"9aa6bb67-c79d-4421-a771-0f032b496522\"}]},\"type\":\"ConnectorPlacement.EquallySpacedConnector\",\"uuid\":\"06545d34-e2f8-440d-8858-488d7d5d7ce4\"}],\"packageUris\":[\"http://schema.mathworks.com/mf0/Connector/R2020b\"],\"version\":\"1.0\"}"
  欠压保护 : Subsystem
      settings: PortSchema="{\"entries\":[{\"content\":{\"headerSize\":26,\"margin\":15,\"minimumSpacing\":25,\"sides\":[{\"content\":{},\"type\":\"ConnectorPlacement.EquallySpacedRectSide\",\"uuid\":\"1beaa6a8-afd1-4db0-ba36-e52cb0b52ffd\"},{\"content\":{\"side\":\"RIGHT\"},\"type\":\"ConnectorPlacement.EquallySpacedRectSide\",\"uuid\":\"b483323e-58d5-432d-ab7d-aadce63dbe6f\"},{\"content\":{\"side\":\"TOP\"},\"type\":\"ConnectorPlacement.EquallySpacedRectSide\",\"uuid\":\"9aa6bb67-c79d-4421-a771-0f032b496522\"}]},\"type\":\"ConnectorPlacement.EquallySpacedConnector\",\"uuid\":\"06545d34-e2f8-440d-8858-488d7d5d7ce4\"}],\"packageUris\":[\"http://schema.mathworks.com/mf0/Connector/R2020b\"],\"version\":\"1.0\"}"
  硬件异常检测 : Subsystem
      settings: PortSchema="{\"entries\":[{\"content\":{\"headerSize\":26,\"margin\":15,\"minimumSpacing\":25,\"sides\":[{\"content\":{},\"type\":\"ConnectorPlacement.EquallySpacedRectSide\",\"uuid\":\"1beaa6a8-afd1-4db0-ba36-e52cb0b52ffd\"},{\"content\":{\"side\":\"RIGHT\"},\"type\":\"ConnectorPlacement.EquallySpacedRectSide\",\"uuid\":\"b483323e-58d5-432d-ab7d-aadce63dbe6f\"},{\"content\":{\"side\":\"TOP\"},\"type\":\"ConnectorPlacement.EquallySpacedRectSide\",\"uuid\":\"9aa6bb67-c79d-4421-a771-0f032b496522\"}]},\"type\":\"ConnectorPlacement.EquallySpacedConnector\",\"uuid\":\"06545d34-e2f8-440d-8858-488d7d5d7ce4\"}],\"packageUris\":[\"http://schema.mathworks.com/mf0/Connector/R2020b\"],\"version\":\"1.0\"}"
  警告检测 : Subsystem
      settings: PortSchema="{\"entries\":[{\"content\":{\"headerSize\":26,\"margin\":15,\"minimumSpacing\":25,\"sides\":[{\"content\":{},\"type\":\"ConnectorPlacement.EquallySpacedRectSide\",\"uuid\":\"1beaa6a8-afd1-4db0-ba36-e52cb0b52ffd\"},{\"content\":{\"side\":\"RIGHT\"},\"type\":\"ConnectorPlacement.EquallySpacedRectSide\",\"uuid\":\"b483323e-58d5-432d-ab7d-aadce63dbe6f\"},{\"content\":{\"side\":\"TOP\"},\"type\":\"ConnectorPlacement.EquallySpacedRectSide\",\"uuid\":\"9aa6bb67-c79d-4421-a771-0f032b496522\"}]},\"type\":\"ConnectorPlacement.EquallySpacedConnector\",\"uuid\":\"06545d34-e2f8-440d-8858-488d7d5d7ce4\"}],\"packageUris\":[\"http://schema.mathworks.com/mf0/Connector/R2020b\"],\"version\":\"1.0\"}"
  过压保护 : Subsystem
      settings: PortSchema="{\"entries\":[{\"content\":{\"headerSize\":26,\"margin\":15,\"minimumSpacing\":25,\"sides\":[{\"content\":{},\"type\":\"ConnectorPlacement.EquallySpacedRectSide\",\"uuid\":\"1beaa6a8-afd1-4db0-ba36-e52cb0b52ffd\"},{\"content\":{\"side\":\"RIGHT\"},\"type\":\"ConnectorPlacement.EquallySpacedRectSide\",\"uuid\":\"b483323e-58d5-432d-ab7d-aadce63dbe6f\"},{\"content\":{\"side\":\"TOP\"},\"type\":\"ConnectorPlacement.EquallySpacedRectSide\",\"uuid\":\"9aa6bb67-c79d-4421-a771-0f032b496522\"}]},\"type\":\"ConnectorPlacement.EquallySpacedConnector\",\"uuid\":\"06545d34-e2f8-440d-8858-488d7d5d7ce4\"}],\"packageUris\":[\"http://schema.mathworks.com/mf0/Connector/R2020b\"],\"version\":\"1.0\"}"
  高温 : Subsystem
      settings: PortSchema="{\"entries\":[{\"content\":{\"headerSize\":26,\"margin\":15,\"minimumSpacing\":25,\"sides\":[{\"content\":{},\"type\":\"ConnectorPlacement.EquallySpacedRectSide\",\"uuid\":\"1beaa6a8-afd1-4db0-ba36-e52cb0b52ffd\"},{\"content\":{\"side\":\"RIGHT\"},\"type\":\"ConnectorPlacement.EquallySpacedRectSide\",\"uuid\":\"b483323e-58d5-432d-ab7d-aadce63dbe6f\"},{\"content\":{\"side\":\"TOP\"},\"type\":\"ConnectorPlacement.EquallySpacedRectSide\",\"uuid\":\"9aa6bb67-c79d-4421-a771-0f032b496522\"}]},\"type\":\"ConnectorPlacement.EquallySpacedConnector\",\"uuid\":\"06545d34-e2f8-440d-8858-488d7d5d7ce4\"}],\"packageUris\":[\"http://schema.mathworks.com/mf0/Connector/R2020b\"],\"version\":\"1.0\"}"

== system servo_hub_task_sys/bsp_init/电流采样校准/从flash里面读取校准值 ==

== system servo_hub_task_sys/bsp_init/电流采样校准/开通pwm校准 ==

== system servo_hub_task_sys/bsp_init/电流采样校准/程序固定值 ==

== system servo_hub_task_sys/bsp_init/编码器初始化/从flash中读取参数配置 ==

== system servo_hub_task_sys/bsp_init/编码器初始化/程序固定值 ==

== system servo_hub_task_sys/pos_ctl_task_10khz/402状态机/PP ==

== system servo_hub_task_sys/pos_ctl_task_10khz/实时安全保护/硬件错误 ==

== system servo_hub_task_sys/pos_ctl_task_10khz/实时安全保护/过流 ==

== system servo_hub_task_sys/pos_ctl_task_10khz/实时安全保护/限位 ==

== system servo_hub_task_sys/task_1ms/电机状态检测/位置误差检测 ==

== system servo_hub_task_sys/task_1ms/电机状态检测/电机堵转检测 ==

== system servo_hub_task_sys/task_1ms/电机状态检测/目标到达检测 ==

== system servo_hub_task_sys/task_1ms/电机状态检测/过速检测 ==

== system servo_hub_task_sys/task_1ms/电机状态检测/零速检测 ==

== system servo_hub_task_sys/task_1ms/非实时安全保护/低温 ==

== system servo_hub_task_sys/task_1ms/非实时安全保护/欠压保护 ==

== system servo_hub_task_sys/task_1ms/非实时安全保护/硬件异常检测 ==

== system servo_hub_task_sys/task_1ms/非实时安全保护/警告检测 ==

== system servo_hub_task_sys/task_1ms/非实时安全保护/过压保护 ==

== system servo_hub_task_sys/task_1ms/非实时安全保护/高温 ==
